simulink model "Simulator_Case_8"  (R2024a)
settings: Solver=VariableStepAuto  StartTime=0.0  StopTime=1400  RelTol=1e-3
values from neighbouring files (symbols this model uses):
  Declination_Sigean = 2.116*(pi/180)    (= 0.0369311669722)    [Parametrization_Simulation_Case_8.m]
  Position_Initial_X = Waypoints_X(1)    [Parametrization_Simulation_Case_8.m]
  Position_Initial_Y = Waypoints_Y(1)    [Parametrization_Simulation_Case_8.m]
  Time_Guidance_Sampling = 20    [Parametrization_Simulation_Case_8.m]
  Time_Period_Sampling = 0.1    [Parametrization_Simulation_Case_8.m]
  Velocity_Norm_Control_Vector = 0    [Velocity_Profile_Norm_Case_8.m]
undefined symbols (not defined in the file or in its folder): Area_Lateral_Projected_Wind, Damping_Coefficient, Damping_Factor_Waves, Density_Air, Density_Water_Salted, Draft_Depth, Drag_Coefficient, Gain_Filter, Inertia_Moment, Length_Ship, Longeron_Area, Mass_Ship, Pulsation_Natural, Pulsation_Wave, Rudder_Angle_Maximal, Rudder_Angle_Minimal, Rudder_Rate_Maximal, Rudder_Rate_Minimal, Static_Gain_Nomoto, Structure_Wind_Coefficient, Time_Constant_Total, Time_Stored, Velocity_Ship_Mean, Waypoints, Yaw_Control_Hydrodynamics_Derivative
libraries: simulink_extras x7, cstblocks x2, sensorinslib x2, sensorgpslib x1
(part 2 of 2)

== matlab function Simulator_Case_8/Environmental_Perturbations/Wind_Perturbation_Torque/Wind_Estimator ==
  data: Wind_Angle_Generated output; Wind_Velocity_Generated output; Wind_Speed output; Velocity_Ship input; Wind_Direction output; Table_Wind_Coefficients input; Yaw_Wind_Coefficient_Current output; Lenght_Ship_Overall input; Density_Air input; Area_Lateral_Projected_Wind input; Inertia_Ship_Vertical_Axis input; Heading_Induced_Wind output; Torque_Wind output; Time_Sampling input
function [Wind_Angle_Generated,...
          Wind_Velocity_Generated,...
          Wind_Speed,...
          Wind_Direction,...
          Yaw_Wind_Coefficient_Current,...
          Heading_Induced_Wind,...
          Torque_Wind] = Wind_Estimator(Velocity_Ship,...
                                        Table_Wind_Coefficients,...
                                        Lenght_Ship_Overall,...
                                        Density_Air,...
                                        Area_Lateral_Projected_Wind,...
                                        Inertia_Ship_Vertical_Axis,...
                                        Time_Sampling)

% Wind estimator and generator online algorithm:
[Wind_Angle_Generated,...
 Wind_Velocity_Generated,...
 Wind_Speed,...
 Wind_Direction,...
 Yaw_Wind_Coefficient_Current,...
 Heading_Induced_Wind,...
 Torque_Wind] = Wind_Estimator_Generator(Velocity_Ship,...
                                         Table_Wind_Coefficients,...
                                         Lenght_Ship_Overall,...
                                         Density_Air,...
                                         Area_Lateral_Projected_Wind,...
                                         Inertia_Ship_Vertical_Axis,...
                                         Time_Sampling);

end

== matlab function Simulator_Case_8/Navigation_And_Wave_Estimator/Wave_Identification_Parameters_ARMA ==
  data: Heading_Wave_High_Frequency_Estimated input; Wave_Pulsation_Estimated output; Wave_Damping_Factor_Estimated output; Time_Sampling input
function [Wave_Pulsation_Estimated,...
          Wave_Damping_Factor_Estimated] = Wave_Parameters_Identification_ARMA(Heading_Wave_High_Frequency_Estimated,...
                                                                               Time_Sampling)

% Two stage Recursive Extended least squares algorithm to estimate the wave
% pulsation and damping factor:
[Wave_Pulsation_Estimated,...
 Wave_Damping_Factor_Estimated] = Wave_Identification_ARMA(Heading_Wave_High_Frequency_Estimated,...
                                                           Time_Sampling);


end

== matlab function Simulator_Case_8/Navigation_And_Wave_Estimator/High_Pass_Filter ==
  data: Heading_Unfiltered_Input input; Heading_Filtered_Ouput output; Time_Sampling input
function Heading_Filtered_Ouput= High_Pass_Wave_Filter(Heading_Unfiltered_Input,...
                                                       Time_Sampling)

% Online numerical high-pass filter for pre-processing of the heading for
% identification:
Heading_Filtered_Ouput = High_Pass_Wave_Filter_Identification(Heading_Unfiltered_Input,...
                                                              Time_Sampling);

end

== matlab function Simulator_Case_8/Ship_Dynamics/Heading_Normalization_Function ==
  data: Heading_Input input; Heading_Normalized output
function Heading_Normalized = Heading_Normalization(Heading_Input)

% This function has the purpose of normalizing the heading angle avoiding
% non-physical values:
Heading_Normalized = mod(Heading_Input, 2*pi);

end

== matlab function Simulator_Case_8/Navigation_And_Wave_Estimator/Sensors_Fusion_And_Filtering/Real_Navigation_Sensors_Extended_Kalman_Filter/INS_Sensor/Velocity_Norm_Calculation ==
  data: Velocity_Input_Vector_Current input; Velocity_Norm_Current output
function Velocity_Norm_Current = Velocity_Norm(Velocity_Input_Vector_Current)

Velocity_Norm_Current = sqrt(Velocity_Input_Vector_Current(1)^2 + Velocity_Input_Vector_Current(2)^2 + Velocity_Input_Vector_Current(3)^2);

end

== matlab function Simulator_Case_8/Controller_And_Actuator/Ship_High_Level_Loop_Controller ==
  data: Heading_Aimed_Current input; Rudder_Angle_Elaborated_Current output; Heading_Observed_Current input; Velocity_Current input; Gain_Filter input; Damping_Aimed input; Pulsation_Aimed input; Time_Sampling input; Length_Ship_Current input; Density_Water_Current input; Drag_Coefficient_Current input; Draft_Depth_Current input; Longeron_Area_Current input; Mass_Of_The_Ship_Current input
function Rudder_Angle_Elaborated_Current = PDF_Controller(Heading_Aimed_Current,...
                                                          Heading_Observed_Current,...
                                                          Velocity_Current,...
                                                          Gain_Filter,...
                                                          Damping_Aimed,...
                                                          Pulsation_Aimed,...
                                                          Time_Sampling,...
                                                          Length_Ship_Current,...
                                                          Density_Water_Current,...
                                                          Drag_Coefficient_Current,...
                                                          Draft_Depth_Current,...
                                                          Longeron_Area_Current,...
                                                          Mass_Of_The_Ship_Current)

% Adaptative control algorithm in function of the velocity:
Rudder_Angle_Elaborated_Current = Controller_PDF_Synthesis_Online_Algorithm(Velocity_Current,...
                                                                            Pulsation_Aimed,...
                                                                            Damping_Aimed,...
                                                                            Gain_Filter,...
                                                                            Length_Ship_Current,...
                                                                            Density_Water_Current,...
                                                                            Drag_Coefficient_Current,...
                                                                            Draft_Depth_Current,...
                                                                            Longeron_Area_Current,...
                                                                            Mass_Of_The_Ship_Current,...
                                                                            Heading_Aimed_Current,...
                                                                            Heading_Observed_Current,...
                                                                            Time_Sampling);

end

== matlab function Simulator_Case_8/Navigation_And_Wave_Estimator/Sensors_Fusion_And_Filtering/Real_Navigation_Sensors_Extended_Kalman_Filter/Heading_Sensor_Fusion_Acceleration ==
  settings: updateMethod=DISCRETE
  data: Position_Ship_X_Current_GPS input; Position_Ship_Y_Current_GPS input; Heading_GPS input; Position_Ship_X_Current_INS input; Position_Ship_Y_Current_INS input; Heading_Current_INS input; Heading_Magnetometer input; Position_Ship_X_Current_Filtered output; Position_Ship_Y_Current_Filtered output; Heading_Ship_Current_Filtered output; Heading_Rate_Current_Filtered output; Velocity_Ship_Mean input; Velocity_Ship_GPS input; Velocity_Ship_INS input; Time_Sampling input; Rudder_Angle_Elaborated input; Bias_Heading_Rate_Current_Model output; Acceleration_INS input; Velocity_Ship_Current output; Acceleration_Ship_Current output; Heading_Rate_INS_Current input; Length_Ship_Current input; Density_Water_Current input; Drag_Coefficient_Current input; Draft_Depth_Current input; Longeron_Area_Current input; Mass_Of_The_Ship_Current input
function [Position_Ship_X_Current_Filtered,...
          Position_Ship_Y_Current_Filtered,...
          Heading_Ship_Current_Filtered,...
          Heading_Rate_Current_Filtered,...
          Bias_Heading_Rate_Current_Model,...
          Velocity_Ship_Current,...
          Acceleration_Ship_Current] = Navigation_Kalman_Sensor_Fusion(Position_Ship_X_Current_GPS,...
                                                                       Position_Ship_Y_Current_GPS,...
                                                                       Heading_GPS,...
                                                                       Position_Ship_X_Current_INS,...
                                                                       Position_Ship_Y_Current_INS,...
                                                                       Heading_Current_INS,...
                                                                       Heading_Magnetometer,...
                                                                       Velocity_Ship_Mean,...
                                                                       Velocity_Ship_GPS,...
                                                                       Velocity_Ship_INS,...
                                                                       Time_Sampling,...
                                                                       Rudder_Angle_Elaborated,...
                                                                       Acceleration_INS,...
                                                                       Heading_Rate_INS_Current,...
                                                                       Length_Ship_Current,...
                                                                       Density_Water_Current,...
                                                                       Drag_Coefficient_Current,...
                                                                       Draft_Depth_Current,...
                                                                       Longeron_Area_Current,...
                                                                       Mass_Of_The_Ship_Current)

% This function serves as a filtering and data fusion to provide the ship
% with the right heading data.
[Position_Ship_X_Current_Filtered,...
 Position_Ship_Y_Current_Filtered,...
 Heading_Ship_Current_Filtered,...
 Heading_Rate_Current_Filtered,...
 Bias_Heading_Rate_Current_Model,...
 Velocity_Ship_Current,...
 Acceleration_Ship_Current] = EKF_Heading_Position_Velocity_Acceleration_Rates(Position_Ship_X_Current_GPS,...
                                                                               Position_Ship_Y_Current_GPS,...
                                                                               Heading_GPS,...
                                                                               Position_Ship_X_Current_INS,...
                                                                               Position_Ship_Y_Current_INS,...
                                                                               Heading_Current_INS,...
                                                                               Heading_Magnetometer,...
                                                                               Velocity_Ship_Mean,...
                                                                               Velocity_Ship_GPS,...
                                                                               Velocity_Ship_INS,...
                                                                               Time_Sampling,...
                                                                               Rudder_Angle_Elaborated,...
                                                                               Acceleration_INS,...
                                                                               Heading_Rate_INS_Current,...
                                                                               Length_Ship_Current,...
                                                                               Density_Water_Current,...
                                                                               Drag_Coefficient_Current,...
                                                                               Draft_Depth_Current,...
                                                                               Longeron_Area_Current,...
                                                                               Mass_Of_The_Ship_Current);



end

== matlab function Simulator_Case_8/Navigation_And_Wave_Estimator/Sensors_Fusion_And_Filtering/Real_Navigation_Sensors_Extended_Kalman_Filter/INS_Sensor/Velocity_Norm_Calculation_INS_Acceleration ==
  data: Velocity_Input_Vector_Current input; Velocity_Norm_Current output
function Velocity_Norm_Current = Velocity_Norm(Velocity_Input_Vector_Current)

% Velocity norm calculation:
Velocity_Norm_Current = sqrt(Velocity_Input_Vector_Current(1)^2 + Velocity_Input_Vector_Current(2)^2 + Velocity_Input_Vector_Current(3)^2);

end

== matlab function Simulator_Case_8/Navigation_And_Wave_Estimator/Sensors_Fusion_And_Filtering/Real_Navigation_Sensors_Extended_Kalman_Filter/INS_Sensor/Acceleration_Norm_Calculation ==
  data: Acceleration_Input_Vector_Current input; Acceleration_Norm_Current output
function Acceleration_Norm_Current = Acceleration_Norm(Acceleration_Input_Vector_Current)

Acceleration_Norm_Current = sqrt(Acceleration_Input_Vector_Current(1)^2 + Acceleration_Input_Vector_Current(2)^2 + Acceleration_Input_Vector_Current(3)^2);

end

== matlab function Simulator_Case_8/Ship_Dynamics/Ship_LPV_Velocity ==
  data: Velocity_Current input; Static_Gain_Nomoto output; Length_Ship_Current input; Density_Water_Current input; Drag_Coefficient_Current input; Draft_Depth_Current input; Longeron_Area_Current input; Mass_Of_The_Ship_Current input; Time_Constant_Total output; Static_Gain_Over_Time output; Inverse_Time output
function [Static_Gain_Nomoto,...
          Time_Constant_Total,...
          Static_Gain_Over_Time,...
          Inverse_Time] = Static_Gain_Time_Constant_Varying_Velocity(Velocity_Current,...
                                                                     Length_Ship_Current,...
                                                                     Density_Water_Current,...
                                                                     Drag_Coefficient_Current,...
                                                                     Draft_Depth_Current,...
                                                                     Longeron_Area_Current,...
                                                                     Mass_Of_The_Ship_Current)


% Only the velocity will be taken into account at first, but all the other terms
% and parameters are considered in inputs for future potential dispersions
% considerations.

% Protection for null velocity declaration:
if Velocity_Current == 0
    Velocity_Current = 5/3.6;
end

% Call of the embedded estimation function:
[Static_Gain_Nomoto,Time_Constant_Total] = Static_Gain_Time_Constant_Varying_Velocity(Velocity_Current,...
                                                                                      Length_Ship_Current,...
                                                                                      Density_Water_Current,...
                                                                                      Drag_Coefficient_Current,...
                                                                                      Draft_Depth_Current,...
                                                                                      Longeron_Area_Current,...
                                                                                      Mass_Of_The_Ship_Current);

% Final operations for LPV Function:
Static_Gain_Over_Time = Static_Gain_Nomoto/Time_Constant_Total;
Inverse_Time = 1/Time_Constant_Total;

end

== matlab function Simulator_Case_8/Guidance_Heading/Guidance_Algorithm ==
  settings: updateMethod=DISCRETE
  data: Velocity_Current input; Heading_Aimed_Next output; Waypoints input; Position_X_Ship_Current input; Position_Y_Ship_Current input; Heading_Ship_Current input; Position_X_Final_Waypoint input; Position_Y_Final_Waypoint input; Time_Current input; Time_End_Guidance output
function [Heading_Aimed_Next,Time_End_Guidance] = Guidance_Waypoints_Following(Velocity_Current,...
                                                                               Waypoints,...
                                                                               Position_X_Ship_Current,...
                                                                               Position_Y_Ship_Current,...
                                                                               Heading_Ship_Current,...
                                                                               Position_X_Final_Waypoint,...
                                                                               Position_Y_Final_Waypoint,...
                                                                               Time_Current)

% Call of the final embedded Guidance function based on Waypoints
% following:
[Heading_Aimed_Next,Time_End_Guidance] = Guidance_Waypoints_Following_Embedded(Velocity_Current,...
                                                                               Waypoints,...
                                                                               Position_X_Ship_Current,...
                                                                               Position_Y_Ship_Current,...
                                                                               Heading_Ship_Current,...
                                                                               Position_X_Final_Waypoint,...
                                                                               Position_Y_Final_Waypoint,...
                                                                               Time_Current);
end

== matlab function Simulator_Case_8/Controller_And_Actuator/Actuator_Control ==
  data: Rudder_Commanded_High_Level_Loop_Current input; Rudder_Commanded_Elaborated_Current output; Rudder_Angle_Maximal input; Rudder_Angle_Minimal input; Rudder_Rate_Maximal input; Rudder_Rate_Minimal input; Time_Sampling input
function Rudder_Commanded_Elaborated_Current = Linear_Actuator_First_Order(Rudder_Commanded_High_Level_Loop_Current,...
                                                                           Rudder_Angle_Maximal,...
                                                                           Rudder_Angle_Minimal,...
                                                                           Rudder_Rate_Maximal,...
                                                                           Rudder_Rate_Minimal,...
                                                                           Time_Sampling)

% This function acts as a simplified model of a first Actuator version. It
% consists in a first saturation of the commanded rudder angle in terms of
% maximal and minimal angles value. And a second saturation in terms of maximal and
% minimal rudder angle rate.
Rudder_Commanded_Elaborated_Current = Rudder_Angle_Rate_Saturations(Rudder_Commanded_High_Level_Loop_Current,...
                                                                    Rudder_Angle_Maximal,...
                                                                    Rudder_Angle_Minimal,...
                                                                    Rudder_Rate_Maximal,...
                                                                    Rudder_Rate_Minimal,...
                                                                    Time_Sampling);

end

== matlab function Simulator_Case_8/Navigation_And_Wave_Estimator/Sensors_Fusion_And_Filtering/Kinematics_Propagator_GPS ==
  settings: updateMethod=DISCRETE
  data: Heading_Angle_Current_Mes input; Position_X_Ship_Init input; Position_Y_Ship_Init input; Time_Simulation_Current input; Position_X_Ship_Compass_Next output; Position_Y_Ship_Compass_Next output; Acceleration_X_Ship_Next output; Acceleration_Y_Ship_Next output; Velocity_X_Ship_Next_Local output; Velocity_Y_Ship_Next_Local output; Time_Sampling input; Velocity_Norm_Current output; Time_Profile_Velocity_Norm input; Velocity_Profile_Norm input
function [Position_X_Ship_Compass_Next,...
          Position_Y_Ship_Compass_Next,...
          Acceleration_X_Ship_Next,...
          Acceleration_Y_Ship_Next,...
          Velocity_X_Ship_Next_Local,...
          Velocity_Y_Ship_Next_Local,...
          Velocity_Norm_Current] = Kinematics_Propagation(Heading_Angle_Current_Mes,...
                                                          Position_X_Ship_Init,...
                                                          Position_Y_Ship_Init,...
                                                          Time_Simulation_Current,...
                                                          Time_Sampling,...
                                                          Time_Profile_Velocity_Norm,...
                                                          Velocity_Profile_Norm)

% Persistents definition:
persistent Position_X_Ship_Compass_Prev
persistent Position_Y_Ship_Compass_Prev
persistent Heading_Previous
persistent Velocity_X_Ship_Local_Previous
persistent Velocity_Y_Ship_Local_Previous

% Heading previous storage:
if isempty(Heading_Previous)
    Heading_Previous = Heading_Angle_Current_Mes;
    Heading_Current = Heading_Previous;
else
    Heading_Current = Heading_Angle_Current_Mes;
end

% Velocity norm based on a predefined profile:
if Time_Simulation_Current == 0 || Time_Simulation_Current < 900
    Velocity_Current = 3/3.6; % Initialization velocity.
elseif Time_Simulation_Current >= 900 && Time_Simulation_Current < 900 + 600
    Velocity_Current = 4/3.6;
elseif Time_Simulation_Current >= 900 + 600 && Time_Simulation_Current < 900 + 600 + 1800
    Velocity_Current = 5/3.6;
elseif Time_Simulation_Current >= 900 + 600 + 1800 && Time_Simulation_Current < 900 + 600 + 1800 + 300
    Velocity_Current = 5/3.6;
else
    Velocity_Current = 3/3.6;
end
Velocity_Norm_Current = Velocity_Current;

% Calculate the local position increment but use both convention (unit and compass):
% Compass:
Position_X_Ship_Current_Increment_Compass = Time_Sampling*Velocity_Norm_Current*sin(Heading_Previous);
Position_Y_Ship_Current_Increment_Compass = Time_Sampling*Velocity_Norm_Current*cos(Heading_Previous);

% The simple velocity discrete increment:
Velocity_X_Ship_Local = Velocity_Norm_Current*sin(Heading_Angle_Current_Mes);
Velocity_Y_Ship_Local = Velocity_Norm_Current*cos(Heading_Angle_Current_Mes);

if isempty(Velocity_X_Ship_Local_Previous)
    Velocity_X_Ship_Local_Previous = Velocity_Norm_Current*sin(Heading_Angle_Current_Mes);
    Acceleration_X_Ship_Next = 0;
else
    Acceleration_X_Ship_Next = (Velocity_X_Ship_Local - Velocity_X_Ship_Local_Previous)/Time_Sampling;
    Velocity_X_Ship_Local_Previous = Velocity_X_Ship_Local;
end
if isempty(Velocity_Y_Ship_Local_Previous)
    Velocity_Y_Ship_Local_Previous = Velocity_Norm_Current*cos(Heading_Angle_Current_Mes);
    Acceleration_Y_Ship_Next = 0;
else
    Acceleration_Y_Ship_Next = (Velocity_Y_Ship_Local - Velocity_Y_Ship_Local_Previous)/Time_Sampling;
    Velocity_Y_Ship_Local_Previous = Velocity_Y_Ship_Local;
end


% Compass position persistent filling:
if isempty(Position_X_Ship_Compass_Prev)
    Position_X_Ship_Compass_Prev = Position_X_Ship_Init + Position_X_Ship_Current_Increment_Compass;
else
    Position_X_Ship_Compass_Prev = Position_X_Ship_Compass_Prev + Position_X_Ship_Current_Increment_Compass;
end
if isempty(Position_Y_Ship_Compass_Prev)
    Position_Y_Ship_Compass_Prev = Position_Y_Ship_Init + Position_Y_Ship_Current_Increment_Compass;
else
    Position_Y_Ship_Compass_Prev = Position_Y_Ship_Compass_Prev + Position_Y_Ship_Current_Increment_Compass;
end

% Then update the outputs:
% Compass:
Position_X_Ship_Compass_Next = Position_X_Ship_Compass_Prev;
Position_Y_Ship_Compass_Next = Position_Y_Ship_Compass_Prev;

% Store the heading:
Heading_Estimated_Next = Heading_Current;
Heading_Previous = Heading_Estimated_Next;

% Velocity:
Velocity_X_Ship_Next_Local = Velocity_X_Ship_Local;
Velocity_Y_Ship_Next_Local = Velocity_Y_Ship_Local;

end
